simulink model "three_phase_pole_diode_with_R_Load"  (R2022a)
settings: Solver=VariableStepAuto  StartTime=0.0  StopTime=0.1  RelTol=1e-3
libraries: spsDiodeLib x6, spsVoltageMeasurementLib x5, spsACVoltageSourceLib x3, spsGroundLib x2, spsCurrentMeasurementLib x1, spsParallelRLCBranchLib x1, spspowerguiLib x1
settings Model: Creator=P.O.M.G  LastModifiedBy=P.O.M.G

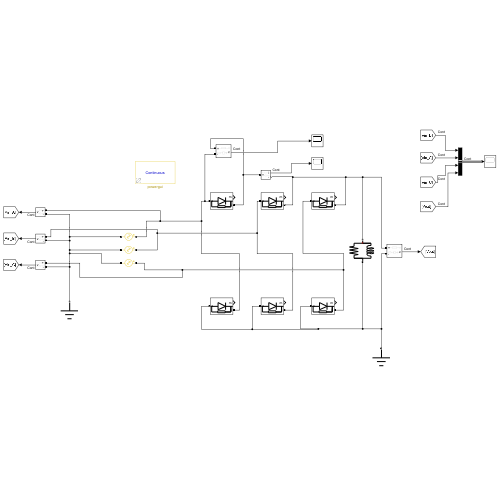
[thumbnail: Simulink's stored preview of the top-level diagram]
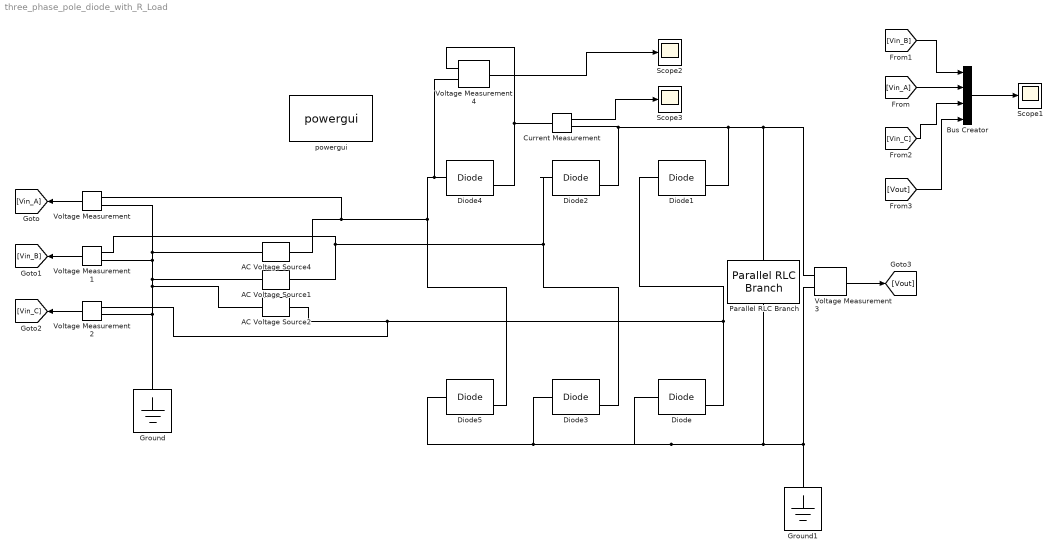
== system three_phase_pole_diode_with_R_Load ==
  AC Voltage Source1 : spsACVoltageSourceLib/AC Voltage Source  Amplitude=308  Phase=120  Frequency=50  SampleTime=1e-5  Measurements=None  BusType=swing  Pref=10e3  Qref=0  Qmin=-inf  Qmax=+inf
  AC Voltage Source2 : spsACVoltageSourceLib/AC Voltage Source  Amplitude=308  Phase=-120  Frequency=50  SampleTime=1e-5  Measurements=None  BusType=swing  Pref=10e3  Qref=0  Qmin=-inf  Qmax=+inf
  AC Voltage Source4 : spsACVoltageSourceLib/AC Voltage Source  Amplitude=308  Phase=0  Frequency=50  SampleTime=1e-5  Measurements=None  BusType=swing  Pref=10e3  Qref=0  Qmin=-inf  Qmax=+inf
  Bus Creator : BusCreator  Inputs=4
  Current Measurement : spsCurrentMeasurementLib/Current Measurement  PhasorSimulation=off  OutputType=Complex  PSBequivalent=0
  Diode{,1..5} (6 alike) : spsDiodeLib/Diode  Ron=0.001  Lon=0  Vf=0.8  IC=0  UseSnubber=0  Rs=500  Cs=250e-9  Measurements=on
  Ground : spsGroundLib/Ground  LConnTagsString=a
  Ground1 : spsGroundLib/Ground  LConnTagsString=a
  Parallel RLC Branch : spsParallelRLCBranchLib/Parallel RLC Branch  LConnTagsString=a  RConnTagsString=__new0  BranchType=RL  Resistance=100  Inductance=2  SetiL0=off  InitialCurrent=0  Capacitance=0  Setx0=off  InitialVoltage=0  Measurements=None
  Scope1 : Scope
  Scope2 : Scope
  Scope3 : Scope
  Voltage Measurement{,1..4} (5 alike) : spsVoltageMeasurementLib/Voltage Measurement  PhasorSimulation=off  OutputType=Complex  PSBequivalent=0
  powergui : spspowerguiLib/powergui  Priority=1  SimulationMode=Continuous  SampleTime=50e-6  frequency=60  Iterations=50  frequencyindice=0  Pbase=100e6  ErrMax=1e-4  UnitsV=kV  UnitsW=MW  buscounter=0  FunctionMessages=off  echomessages=off  EnableUseOfTLC=off  CurrentSourceSwitches=off  DisableSnubberDevices=off  DisableRonSwitches=off  DisableVfSwitches=off  DisplayEquations=off  AutomaticDiscreteSolvers=off  SolverType=Tustin/Backward Euler (TBE)  Interpol=off  ExternalGateDelay=off  methode=off  Ts=100  x0status=blocks  SPID=on  SwTol=0  HookPort=off  NonlinearTolerance=1e-4  nMaxIteration=100  ContinueOnMaxIteration=off  RestoreLinks=warning  ResistiveCurrentMeasurement=off  Frange=[0:2:500]  Ylog=off  Xlog=on  ShowGrid=off  save=off  variable=ZData  structure=0  ZoomFFT=off  StartTime=0.0  cycles=1  DisplayStyle=1  fundamental=60  FreqAxis=off  MaxFrequency=1000  frequencyindicesteady=1  RmsSteady=1  display=off
  wires:
  Voltage Measurement2/1 -> [Vin_C]
  Voltage Measurement1/1 -> [Vin_B]
  Voltage Measurement/1 -> [Vin_A]
  [Vin_B] -> Bus Creator/1
  [Vin_A] -> Bus Creator/2
  [Vin_C] -> Bus Creator/3
  [Vout] -> Bus Creator/4
  Bus Creator/1 -> Scope1/1
  Voltage Measurement3/1 -> [Vout]
  Voltage Measurement4/1 -> Scope2/1
  Current Measurement/1 -> Scope3/1
  connections:
  Ground/LConn1 -- AC Voltage Source2/LConn1 -- AC Voltage Source4/LConn1 -- Voltage Measurement/LConn2 -- Voltage Measurement1/LConn2 -- AC Voltage Source1/LConn1 -- Voltage Measurement2/LConn2
  Diode/LConn1 -- Ground1/LConn1 -- Voltage Measurement3/LConn2 -- Parallel RLC Branch/RConn1 -- Diode5/LConn1 -- Diode3/LConn1
  Diode2/RConn1 -- Parallel RLC Branch/LConn1 -- Voltage Measurement3/LConn1 -- Diode1/RConn1 -- Current Measurement/RConn1
  Diode4/LConn1 -- Voltage Measurement4/LConn2 -- AC Voltage Source4/RConn1 -- Voltage Measurement/LConn1 -- Diode5/RConn1
  Diode2/LConn1 -- AC Voltage Source1/RConn1 -- Voltage Measurement1/LConn1 -- Diode3/RConn1
  Diode1/LConn1 -- AC Voltage Source2/RConn1 -- Voltage Measurement2/LConn1 -- Diode/RConn1
  Voltage Measurement4/LConn1 -- Diode4/RConn1 -- Current Measurement/LConn1
